simulink model "TSMCDTC"  (R2016b)
settings: Solver=VariableStepAuto  StartTime=0.0  StopTime=1  RelTol=1e-3  EnableMultiTasking=on
model workspace (MAT data in the model file):
  Cf = 1e-05
  J = 0.02
  Lf = 0.005
  Lm = 0.27325
  Lr = 0.289368
  Ls = 0.289368
  P = 4
  Rf = 5
  Rr = 3.3278
  Rs = 4.6
  theta0 = 0
undefined symbols (not defined in the file or in its folder): magnitude
libraries: powerlib x35, simulink x3
settings Model: PauseTimes=0.0143  Creator=yoush  LastModifiedBy=itsys
settings DataIOCC: LimitDataPoints=on  SaveFormat=Array
settings OptimizationCC: LifeSpan=inf
settings DebuggingCC: UnderspecifiedInitializationDetection=Classic  MergeDetectMultiDrivingBlocksExec=none  SolverPrmCheckMsg=warning  AllowSymbolicDim=off  SFUnexpectedBacktrackingDiag=warning  SFNoUnconditionalDefaultTransitionDiag=warning  SFExecutionAtInitializationDiag=none
settings HardwareCC: ProdBitPerPointer=32  ProdBitPerSizeT=32  ProdBitPerPtrDiffT=32  ProdLargestAtomicFloat=None  ProdIntDivRoundTo=Undefined  ProdEndianess=Unspecified  ProdWordSize=32  ProdHWDeviceType=32-bit Generic
settings ModelReferenceCC: PropagateSignalLabelsOutOfModel=off
settings GRTTargetCC: TargetLangStandard=C89/C90 (ANSI)  GeneratePreprocessorConditionals=Disable all
settings ConfigComp: CovMetricSettings=dw  CovHtmlReporting=on  CovSaveCumulativeToWorkspaceVar=on  CovSaveSingleToWorkspaceVar=on  CovExternalEMLEnable=off

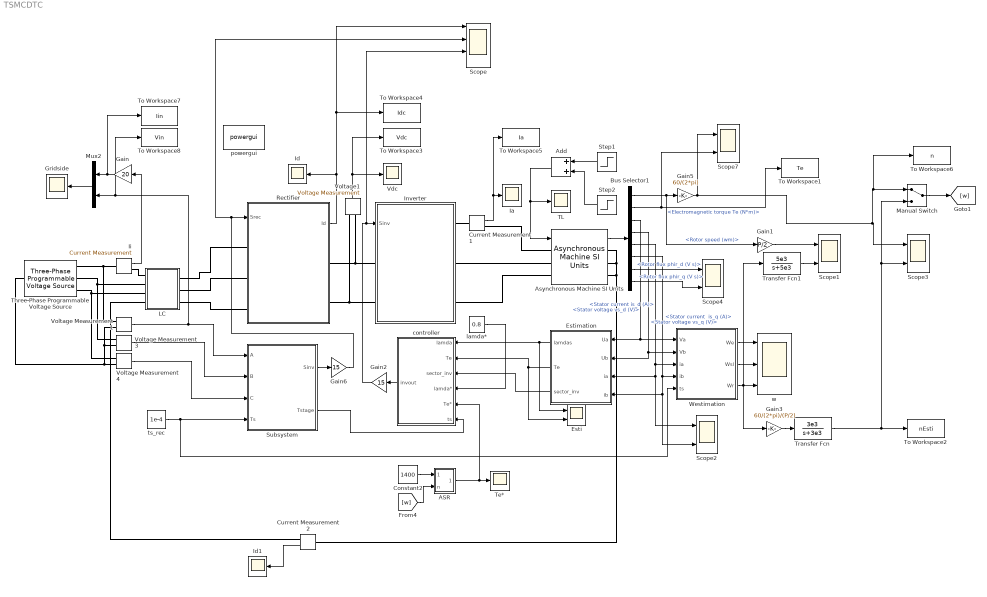
== system TSMCDTC ==
  ASR : Subsystem
  Add : Sum
  Asynchronous Machine SI Units : powerlib/Machines/Asynchronous Machine SI Units  RotorType=Wound  PresetModel=No  MechanicalLoad=Torque Tm  ShowDetailedParameters=on  ReferenceFrame=Stationary  Units=SI  MeasurementBus=off  NominalParameters=[22000 380 50]  Stator=[4.6 0.016118]  Rotor=[3.3278 0.016118]  Cage1=[0.4155 0.002066]  Cage2=[0.4168 0.0003495]  Lm=0.27325  Mechanical=[0.02 0 2]  PolePairs=2  InitialConditions=[ 1 0 0 0 0 0 0 0]  SimulateSaturation=off  Saturation=[14.03593122, 27.81365428, 53.79336849, 72.68890987, 97.98006896, 148.6815601, 215.7428561, 302.9841135, 428.7778367 ; 230, 322, 414, 460, 506, 552, 598, 644, 690]  LoadFlowParameters=1492000  TsPowergui=0  TsBlock=-1  IterativeModel=Trapezoidal non iterative  IterativeDiscreteModel=Trapezoidal non iterative  Pmec=1.492e+006
  Bus Selector1 : BusSelector  OutputSignals="Mechanical.Rotor speed (wm),Mechanical.Electromagnetic torque Te (N*m),Stator measurements.Stator voltage vs_d (V),Stator measurements.Stator voltage vs_q (V),Stator measurements.Stator current is_d (A),Stator measurements.Stator current  is_q (A),Rotor measurements.Rotor flux phir_d (V s),Rotor measurements.Rotor flux phir_q (V s)"
  Constant2 : Constant  Value=1400
  Current Measurement1 : powerlib/Measurements/Current Measurement  PhasorSimulation=off  OutputType=Complex  PSBequivalent=0
  Current Measurement2 : powerlib/Measurements/Current Measurement  PhasorSimulation=off  OutputType=Complex  PSBequivalent=0
  Esti : Scope  NumInputPorts=2
  Estimation : Subsystem
  Gain : Gain  Gain=20
  Gain1 : Gain  Gain=P/2
  Gain2 : Gain  Gain=15
  Gain3 : Gain  Gain=60/(2*pi)/(P/2)
  Gain5 : Gain  Gain=60/(2*pi)
  Gain6 : Gain  Gain=15
  Gridside : Scope
  Ia : Scope
  Id : Scope
  Id1 : Scope
  Ii : powerlib/Measurements/Current Measurement  PhasorSimulation=off  OutputType=Complex  PSBequivalent=0
  Inverter : Subsystem
  LC : Subsystem
  Manual Switch : ManualSwitch
  Mux2 : Mux  Inputs=2
  Rectifier : Subsystem
  Scope : Scope  NumInputPorts=4
  Scope{1..4,7} (5 alike) : Scope  NumInputPorts=2
  Step1 : Step  Time=0.4  After=5  SampleTime=0
  Step2 : Step  Time=0.7  After=5  SampleTime=0
  Subsystem : Subsystem
  TL : Scope
  Te* : Scope
  Three-Phase Programmable Voltage Source : powerlib/Electrical Sources/Three-Phase Programmable Voltage Source  PositiveSequence="[380  0 50]"  VariationEntity=None  VariationType=Table of time-amplitude pairs  VariationTypeAlt=Step  VariationStep=0.5  VariationRate=10  VariationMagnitude=0.3  VariationFrequency=2  VariationTiming=[1 2]  VariationPhaseA=off  Amplitudes=[1 0.8 1.2 1.0]  TimeValues=[0 0.1 0.15 0.2]  HarmonicGeneration=off  HarmonicA=[3 0.2 -25 0]  HarmonicB=[2 0.15 35 2]  Timing="[0.05  3]"  BusType=swing  Pref=0  Qref=0  Qmin=-inf  Qmax=inf
  To Workspace1 : ToWorkspace  VariableName=Te  SaveFormat=Timeseries  SampleTime=-1
  To Workspace2 : ToWorkspace  VariableName=nEsti  SaveFormat=Timeseries  SampleTime=-1
  To Workspace3 : ToWorkspace  VariableName=Vdc  SaveFormat=Timeseries  SampleTime=-1
  To Workspace4 : ToWorkspace  VariableName=Idc  SaveFormat=Timeseries  SampleTime=-1
  To Workspace5 : ToWorkspace  VariableName=Ia  SaveFormat=Timeseries  SampleTime=-1
  To Workspace6 : ToWorkspace  VariableName=n  SaveFormat=Timeseries  SampleTime=-1
  To Workspace7 : ToWorkspace  VariableName=Iin  SaveFormat=Timeseries  SampleTime=-1
  To Workspace8 : ToWorkspace  VariableName=Vin  SaveFormat=Timeseries  SampleTime=-1
  Transfer Fcn : TransferFcn  Numerator=[3e3]  Denominator=[1 3e3]
  Transfer Fcn1 : TransferFcn  Numerator=[5e3]  Denominator=[1 5e3]
  Vdc : Scope
  Voltage Measurement1 : powerlib/Measurements/Voltage Measurement  PhasorSimulation=off  OutputType=Complex  PSBequivalent=0
  Voltage Measurement3 : powerlib/Measurements/Voltage Measurement  PhasorSimulation=off  OutputType=Complex  PSBequivalent=0
  Voltage Measurement4 : powerlib/Measurements/Voltage Measurement  PhasorSimulation=off  OutputType=Complex  PSBequivalent=0
  Voltage1 : powerlib/Measurements/Voltage Measurement  PhasorSimulation=off  OutputType=Complex  PSBequivalent=0
  Westimation : Subsystem
  controller : Subsystem
  lamda* : Constant  Value=0.8
  powergui : powerlib/powergui  Priority=1  SimulationMode=Continuous  SolverType=Tustin  SampleTime=5e-7  frequency=60  SPID=off  DisableSnubberDevices=off  DisableRonSwitches=off  DisableVfSwitches=off  SwTol=0  DisplayEquations=off  Interpol=off  ExternalGateDelay=off  methode=off  Ts=0  FunctionMessages=off  echomessages=off  HookPort=off  EnableUseOfTLC=off  x0status=blocks  frequencyindice=50  Pbase=100e6  ErrMax=1e-4  Iterations=50  UnitsV=kV  UnitsW=MW  buscounter=0  RestoreLinks=warning  ResistiveCurrentMeasurement=off  Frange=[0:2:500]  Ylog=off  Xlog=on  ShowGrid=off  save=off  variable=ZData  structure=input  ZoomFFT=off  StartTime=0.5  cycles=5  DisplayStyle=1  fundamental=50  FreqAxis=off  MaxFrequency=10000  frequencyindicesteady=1  RmsSteady=1  display=off
  ts_rec : Constant  Value=1e-4
  w : Scope  NumInputPorts=3
  wires:
  Current Measurement1/1 -> To Workspace5/1, Ia/1
  Asynchronous Machine SI Units/1 -> Bus Selector1/1
  Bus Selector1/2 -> Scope7/2, To Workspace1/1  "<Electromagnetic torque Te (N*m)>"
  Bus Selector1/1 -> Gain1/1, Gain5/1  "<Rotor speed (wm)>"
  Bus Selector1/3 -> Estimation/1(Ua), Westimation/1(Va)  "<Stator voltage vs_d (V)>"
  Step1/1 -> Add/1
  Step2/1 -> Add/2
  Add/1 -> Asynchronous Machine SI Units/1, TL/1
  lamda*/1 -> controller/4(lamda*)
  controller/1(invout) -> Gain2/1
  Gain5/1 -> To Workspace6/1, Manual Switch/1, Scope3/1, Scope7/1
  Gain6/1 -> Scope/2, Rectifier/1(Srec)
  Rectifier/1(Id) -> Scope/1, To Workspace4/1, Id/1
  Gain2/1 -> Scope/3, Inverter/1(Sinv)
  Westimation/1(We) -> w/1
  Westimation/2(Wsl) -> w/2
  Bus Selector1/4 -> Westimation/2(Vb), Estimation/2(Ub)  "<Stator voltage vs_q (V)>"
  Bus Selector1/5 -> Westimation/3(ia), Scope2/1, Estimation/3(ia)  "<Stator current is_d (A)>"
  Bus Selector1/6 -> Westimation/4(ib), Scope2/2, Estimation/4(ib)  "<Stator current  is_q (A)>"
  Estimation/1(lamdas) -> Esti/1, controller/1(lamda)
  Estimation/2(Te) -> Esti/2, controller/2(Te)
  Estimation/3(sector_inv) -> controller/3(sector_inv)
  Voltage Measurement1/1 -> To Workspace8/1, Mux2/2, Subsystem/1(A)
  Voltage Measurement3/1 -> Subsystem/2(B)
  Voltage Measurement4/1 -> Subsystem/3(C)
  Subsystem/1(Sinv) -> Gain6/1
  Voltage1/1 -> Vdc/1, To Workspace3/1
  Mux2/1 -> Gridside/1
  Ii/1 -> Gain/1
  Gain1/1 -> Scope1/1
  Gain3/1 -> Transfer Fcn/1
  Westimation/3(Wr) -> Transfer Fcn1/1, Gain3/1, w/3
  Transfer Fcn1/1 -> Scope1/2
  Transfer Fcn/1 -> To Workspace2/1, Manual Switch/2, Scope3/2
  Manual Switch/1 -> [w]
  Bus Selector1/7 -> Scope4/1  "<Rotor flux phir_d (V s)>"
  Bus Selector1/8 -> Scope4/2  "<Rotor flux phir_q (V s)>"
  ASR/1(Te*) -> Te*/1, controller/5(Te*)
  Constant2/1 -> ASR/1(n*)
  [w] -> ASR/2(n)
  ts_rec/1 -> Westimation/5(ts), Subsystem/4(Ts)
  Subsystem/2(Tstage) -> controller/6(ts)
  Gain/1 -> To Workspace7/1, Mux2/1
  Current Measurement2/1 -> Id1/1
  connections:
  Voltage Measurement1/LConn1 -- Three-Phase Programmable Voltage Source/RConn1 -- Ii/LConn1
  Three-Phase Programmable Voltage Source/LConn1 -- Voltage Measurement1/LConn2 -- Voltage Measurement3/LConn2 -- Voltage Measurement4/LConn2
  Current Measurement1/RConn1 -- Asynchronous Machine SI Units/LConn1
  Current Measurement1/LConn1 -- Inverter/RConn1
  Asynchronous Machine SI Units/LConn2 -- Inverter/RConn2
  Asynchronous Machine SI Units/LConn3 -- Inverter/RConn3
  Rectifier/RConn1 -- Inverter/LConn1 -- Voltage1/LConn1
  Rectifier/RConn2 -- Inverter/LConn2 -- Voltage1/LConn2
  Voltage Measurement3/LConn1 -- Three-Phase Programmable Voltage Source/RConn2 -- LC/LConn2
  Three-Phase Programmable Voltage Source/RConn3 -- LC/LConn3 -- Voltage Measurement4/LConn1
  LC/LConn1 -- Ii/RConn1
  LC/RConn1 -- Rectifier/LConn1
  LC/RConn2 -- Rectifier/LConn2
  LC/RConn3 -- Rectifier/LConn3
  Asynchronous Machine SI Units/RConn2 -- Current Measurement2/LConn1 -- Asynchronous Machine SI Units/RConn3 -- Asynchronous Machine SI Units/RConn1
  Current Measurement2/RConn1 -- LC/LConn4

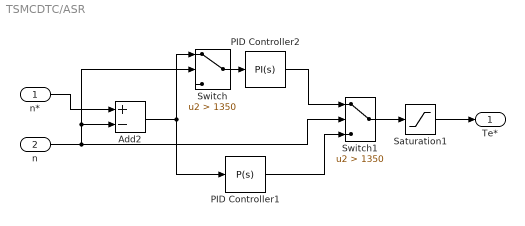
== system TSMCDTC/ASR ==
  n* : Inport
  n : Inport  Port=2
  Add2 : Sum  Inputs=+-
  PID Controller1 : simulink/Continuous/PID Controller  Controller=P  TimeDomain=Continuous-time  SampleTime=-1  IntegratorMethod=Forward Euler  FilterMethod=Forward Euler  Form=Parallel  UseFilter=on  ControllerParametersSource=internal  P=1  I=0  D=0  N=100  InitialConditionSource=internal  InitialConditionForIntegrator=0  InitialConditionForFilter=0  ExternalReset=none  LimitOutput=off  UpperSaturationLimit=inf  LowerSaturationLimit=-inf  LinearizeAsGain=on  AntiWindupMode=none  Kb=1  TrackingMode=off  Kt=1  PParamMin=[]  PParamMax=[]  IParamMin=[]  IParamMax=[]  DParamMin=[]  DParamMax=[]  NParamMin=[]  NParamMax=[]  KbParamMin=[]  KbParamMax=[]  KtParamMin=[]  KtParamMax=[]  POutMin=[]  POutMax=[]  IOutMin=[]  IOutMax=[]  DOutMin=[]  DOutMax=[]  NOutMin=[]  NOutMax=[]  KbOutMin=[]  KbOutMax=[]  KtOutMin=[]  KtOutMax=[]  IntegratorOutMin=[]  IntegratorOutMax=[]  FilterOutMin=[]  FilterOutMax=[]  SumOutMin=[]  SumOutMax=[]  SumI1OutMin=[]  SumI1OutMax=[]  SumI2OutMin=[]  SumI2OutMax=[]  SumI3OutMin=[]  SumI3OutMax=[]  SumDOutMin=[]  SumDOutMax=[]  SaturationOutMin=[]  SaturationOutMax=[]  IntegratorContinuousStateAttributes=''  IntegratorStateMustResolveToSignalObject=off  IntegratorRTWStateStorageClass=Auto  FilterContinuousStateAttributes=''  FilterStateMustResolveToSignalObject=off  FilterRTWStateStorageClass=Auto  DifferentiatorICPrevScaledInput=0  DifferentiatorOutMin=[]  DifferentiatorOutMax=[]
  PID Controller2 : simulink/Continuous/PID Controller  Controller=PI  TimeDomain=Continuous-time  SampleTime=-1  IntegratorMethod=Forward Euler  FilterMethod=Forward Euler  Form=Parallel  UseFilter=on  ControllerParametersSource=internal  P=0.3  I=30  D=0  N=100  InitialConditionSource=internal  InitialConditionForIntegrator=0  InitialConditionForFilter=0  ExternalReset=none  LimitOutput=off  UpperSaturationLimit=inf  LowerSaturationLimit=-inf  LinearizeAsGain=on  AntiWindupMode=none  Kb=1  TrackingMode=off  Kt=1  PParamMin=[]  PParamMax=[]  IParamMin=[]  IParamMax=[]  DParamMin=[]  DParamMax=[]  NParamMin=[]  NParamMax=[]  KbParamMin=[]  KbParamMax=[]  KtParamMin=[]  KtParamMax=[]  POutMin=[]  POutMax=[]  IOutMin=[]  IOutMax=[]  DOutMin=[]  DOutMax=[]  NOutMin=[]  NOutMax=[]  KbOutMin=[]  KbOutMax=[]  KtOutMin=[]  KtOutMax=[]  IntegratorOutMin=[]  IntegratorOutMax=[]  FilterOutMin=[]  FilterOutMax=[]  SumOutMin=[]  SumOutMax=[]  SumI1OutMin=[]  SumI1OutMax=[]  SumI2OutMin=[]  SumI2OutMax=[]  SumI3OutMin=[]  SumI3OutMax=[]  SumDOutMin=[]  SumDOutMax=[]  SaturationOutMin=[]  SaturationOutMax=[]  IntegratorContinuousStateAttributes=''  IntegratorStateMustResolveToSignalObject=off  IntegratorRTWStateStorageClass=Auto  FilterContinuousStateAttributes=''  FilterStateMustResolveToSignalObject=off  FilterRTWStateStorageClass=Auto  DifferentiatorICPrevScaledInput=0  DifferentiatorOutMin=[]  DifferentiatorOutMax=[]
  Saturation1 : Saturate  UpperLimit=15  LowerLimit=-15
  Switch : Switch  Criteria=u2 > Threshold  Threshold=1350
  Switch1 : Switch  Criteria=u2 > Threshold  Threshold=1350
  Te* : Outport
  wires:
  Saturation1/1 -> Te*/1
  PID Controller1/1 -> Switch1/3
  Switch1/1 -> Saturation1/1
  PID Controller2/1 -> Switch1/1
  Switch/1 -> PID Controller2/1
  Add2/1 -> PID Controller1/1, Switch/1
  n*/1 -> Add2/1
  n/1 -> Switch1/2, Switch/2, Add2/2

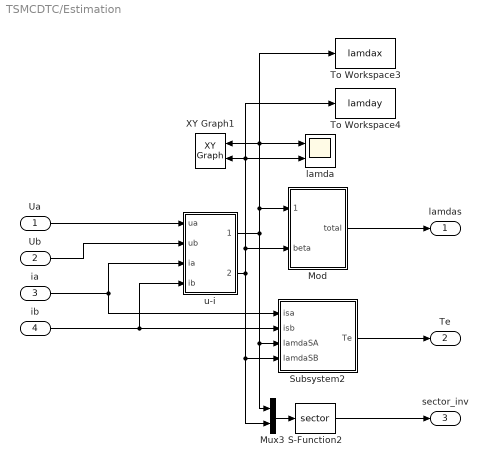
== system TSMCDTC/Estimation ==
  Ua : Inport
  Ub : Inport  Port=2
  ia : Inport  Port=3
  ib : Inport  Port=4
  Mod : Subsystem
  Mux3 : Mux  Inputs=2
  S-Function2 : S-Function  FunctionName=sector  SFunctionDeploymentMode=off  EnableBusSupport=off
  Subsystem2 : Subsystem
  To Workspace3 : ToWorkspace  VariableName=lamdax  SaveFormat=Timeseries  SampleTime=-1
  To Workspace4 : ToWorkspace  VariableName=lamday  SaveFormat=Timeseries  SampleTime=-1
  XY Graph1 : simulink/Sinks/XY Graph  xmin=-1.5  xmax=1.5  ymin=-1.5  ymax=1.5  st=-1
  lamda : Scope  NumInputPorts=2
  u-i : Subsystem
  lamdas : Outport
  Te : Outport  Port=2
  sector_inv : Outport  Port=3
  wires:
  u-i/1(lamdaSA) -> Mux3/1, Subsystem2/3(lamdaSA), To Workspace3/1, lamda/1, XY Graph1/1, Mod/1(alpha)
  u-i/2(lamdaSB) -> Mux3/2, Subsystem2/4(lamdaSB), To Workspace4/1, lamda/2, XY Graph1/2, Mod/2(beta)
  Mux3/1 -> S-Function2/1
  Ua/1 -> u-i/1(ua)
  Ub/1 -> u-i/2(ub)
  ia/1 -> u-i/3(ia), Subsystem2/1(isa)
  ib/1 -> u-i/4(ib), Subsystem2/2(isb)
  S-Function2/1 -> sector_inv/1
  Subsystem2/1(Te) -> Te/1
  Mod/1(total) -> lamdas/1

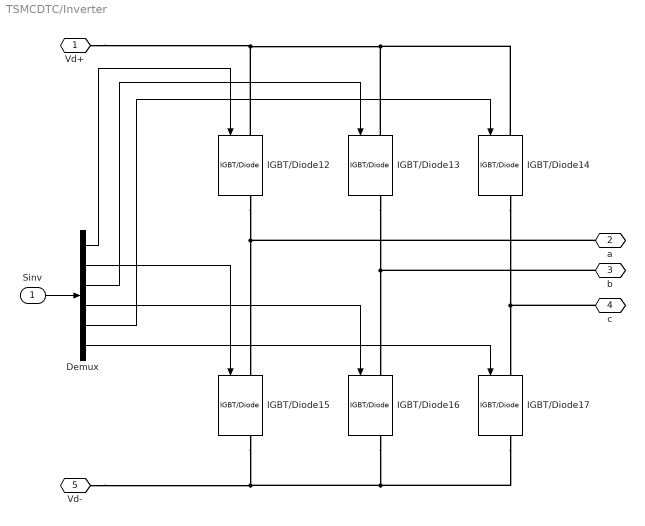
== system TSMCDTC/Inverter ==
  Sinv : Inport
  Demux : Demux  Outputs=6
  IGBT/Diode{12..17} (6 alike) : powerlib/Power Electronics/IGBT//Diode  Ron=1e-3  Rs=1e5  Cs=inf  Measurements=on
  Vd+ : PMIOPort  Port=1  Side=Left
  a : PMIOPort  Port=2  Side=Right
  b : PMIOPort  Port=3  Side=Right
  c : PMIOPort  Port=4  Side=Right
  Vd- : PMIOPort  Port=5  Side=Left
  wires:
  Demux/5 -> IGBT/Diode14/1
  Demux/4 -> IGBT/Diode16/1
  Demux/3 -> IGBT/Diode13/1
  Demux/6 -> IGBT/Diode17/1
  Demux/1 -> IGBT/Diode12/1
  Sinv/1 -> Demux/1
  Demux/2 -> IGBT/Diode15/1
  connections:
  IGBT/Diode12/RConn1 -- IGBT/Diode15/LConn1 -- a/RConn1
  IGBT/Diode13/RConn1 -- IGBT/Diode16/LConn1 -- b/RConn1
  IGBT/Diode14/RConn1 -- IGBT/Diode17/LConn1 -- c/RConn1
  IGBT/Diode17/RConn1 -- IGBT/Diode16/RConn1 -- Vd-/RConn1 -- IGBT/Diode15/RConn1
  IGBT/Diode12/LConn1 -- Vd+/RConn1 -- IGBT/Diode13/LConn1 -- IGBT/Diode14/LConn1

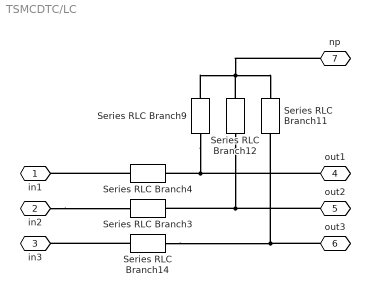
== system TSMCDTC/LC ==
  Series RLC Branch11 : powerlib/Elements/Series RLC Branch  LConnTagsString=__new0  RConnTagsString=__new0  BranchType=C  Resistance=1  Inductance=0.5e-3  SetiL0=off  InitialCurrent=0  Capacitance=Cf  Setx0=off  InitialVoltage=0  Measurements=None
  Series RLC Branch12 : powerlib/Elements/Series RLC Branch  LConnTagsString=__new0  RConnTagsString=__new0  BranchType=C  Resistance=1  Inductance=0.5e-3  SetiL0=off  InitialCurrent=0  Capacitance=Cf  Setx0=off  InitialVoltage=0  Measurements=None
  Series RLC Branch14 : powerlib/Elements/Series RLC Branch  LConnTagsString=__new0  RConnTagsString=__new0  BranchType=RL  Resistance=Rf  Inductance=Lf  SetiL0=off  InitialCurrent=0  Capacitance=1e-6  Setx0=off  InitialVoltage=0  Measurements=None
  Series RLC Branch3 : powerlib/Elements/Series RLC Branch  LConnTagsString=__new0  RConnTagsString=__new0  BranchType=RL  Resistance=Rf  Inductance=Lf  SetiL0=off  InitialCurrent=0  Capacitance=1e-6  Setx0=off  InitialVoltage=0  Measurements=None
  Series RLC Branch4 : powerlib/Elements/Series RLC Branch  LConnTagsString=__new0  RConnTagsString=__new0  BranchType=RL  Resistance=Rf  Inductance=Lf  SetiL0=off  InitialCurrent=0  Capacitance=1e-6  Setx0=off  InitialVoltage=0  Measurements=None
  Series RLC Branch9 : powerlib/Elements/Series RLC Branch  LConnTagsString=__new0  RConnTagsString=__new0  BranchType=C  Resistance=1  Inductance=0.5e-3  SetiL0=off  InitialCurrent=0  Capacitance=Cf  Setx0=off  InitialVoltage=0  Measurements=None
  in1 : PMIOPort  Port=1  Side=Left
  in2 : PMIOPort  Port=2  Side=Left
  in3 : PMIOPort  Port=3  Side=Left
  out1 : PMIOPort  Port=4  Side=Right
  out2 : PMIOPort  Port=5  Side=Right
  out3 : PMIOPort  Port=6  Side=Right
  np : PMIOPort  Port=7  Side=Left
  connections:
  Series RLC Branch4/LConn1 -- in1/RConn1
  Series RLC Branch14/LConn1 -- in3/RConn1
  in2/RConn1 -- Series RLC Branch3/LConn1
  Series RLC Branch9/RConn1 -- np/RConn1 -- Series RLC Branch12/RConn1 -- Series RLC Branch11/RConn1
  out1/RConn1 -- Series RLC Branch9/LConn1 -- Series RLC Branch4/RConn1
  out2/RConn1 -- Series RLC Branch12/LConn1 -- Series RLC Branch3/RConn1
  Series RLC Branch14/RConn1 -- out3/RConn1 -- Series RLC Branch11/LConn1

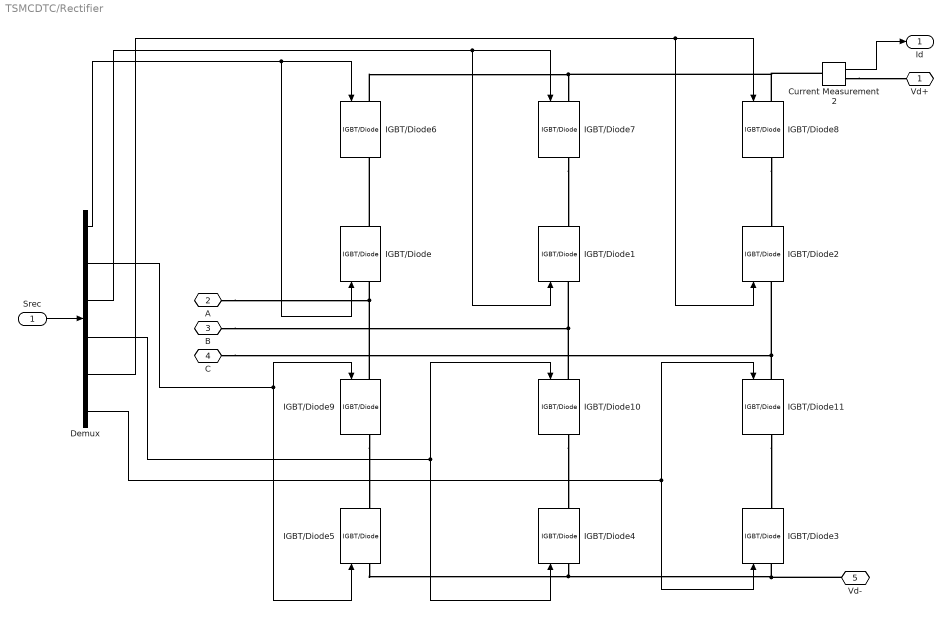
== system TSMCDTC/Rectifier ==
  Srec : Inport
  Current Measurement2 : powerlib/Measurements/Current Measurement  PhasorSimulation=off  OutputType=Complex  PSBequivalent=0
  Demux : Demux  Outputs=6
  IGBT/Diode{,1..11} (12 alike) : powerlib/Power Electronics/IGBT//Diode  Ron=1e-3  Rs=1e5  Cs=inf  Measurements=on
  Vd+ : PMIOPort  Port=1  Side=Right
  A : PMIOPort  Port=2  Side=Left
  B : PMIOPort  Port=3  Side=Left
  "C " : PMIOPort  Port=4  Side=Left
  Vd- : PMIOPort  Port=5  Side=Right
  Id : Outport
  wires:
  Srec/1 -> Demux/1
  Demux/1 -> IGBT/Diode/1, IGBT/Diode6/1
  Demux/2 -> IGBT/Diode5/1, IGBT/Diode9/1
  Demux/3 -> IGBT/Diode1/1, IGBT/Diode7/1
  Demux/5 -> IGBT/Diode8/1, IGBT/Diode2/1
  Demux/4 -> IGBT/Diode10/1, IGBT/Diode4/1
  Demux/6 -> IGBT/Diode3/1, IGBT/Diode11/1
  Current Measurement2/1 -> Id/1
  connections:
  IGBT/Diode11/RConn1 -- IGBT/Diode3/RConn1
  IGBT/Diode10/RConn1 -- IGBT/Diode4/RConn1
  IGBT/Diode8/RConn1 -- IGBT/Diode2/RConn1
  IGBT/Diode9/RConn1 -- IGBT/Diode5/RConn1
  IGBT/Diode9/LConn1 -- A/RConn1 -- IGBT/Diode/LConn1
  IGBT/Diode6/LConn1 -- IGBT/Diode8/LConn1 -- Current Measurement2/LConn1 -- IGBT/Diode7/LConn1
  IGBT/Diode7/RConn1 -- IGBT/Diode1/RConn1
  IGBT/Diode/RConn1 -- IGBT/Diode6/RConn1
  IGBT/Diode10/LConn1 -- B/RConn1 -- IGBT/Diode1/LConn1
  IGBT/Diode11/LConn1 -- "C "/RConn1 -- IGBT/Diode2/LConn1
  IGBT/Diode5/LConn1 -- IGBT/Diode4/LConn1 -- Vd-/RConn1 -- IGBT/Diode3/LConn1
  Current Measurement2/RConn1 -- Vd+/RConn1

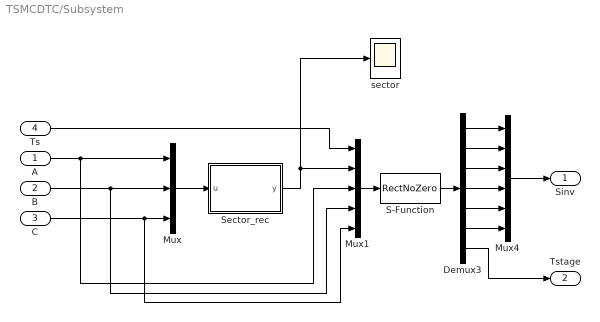
== system TSMCDTC/Subsystem ==
  A : Inport
  B : Inport  Port=2
  C : Inport  Port=3
  Ts : Inport  Port=4
  Demux3 : Demux  Outputs=7
  Mux : Mux  Inputs=3
  Mux1 : Mux  Inputs=5
  Mux4 : Mux  Inputs=6
  S-Function : S-Function  FunctionName=RectNoZero  SFunctionDeploymentMode=off  EnableBusSupport=off
  Sector_rec : MATLAB Function  TreatAsAtomicUnit=on
  sector : Scope
  Sinv : Outport
  Tstage : Outport  Port=2
  wires:
  B/1 -> Mux/2, Mux1/4
  Mux/1 -> Sector_rec/1(u)
  A/1 -> Mux/1, Mux1/3
  Sector_rec/1(y) -> Mux1/2, sector/1
  C/1 -> Mux1/5, Mux/3
  Demux3/5 -> Mux4/5
  Demux3/6 -> Mux4/6
  Demux3/2 -> Mux4/2
  Demux3/1 -> Mux4/1
  Mux4/1 -> Sinv/1
  S-Function/1 -> Demux3/1
  Demux3/4 -> Mux4/4
  Demux3/3 -> Mux4/3
  Mux1/1 -> S-Function/1
  Ts/1 -> Mux1/1
  Demux3/7 -> Tstage/1

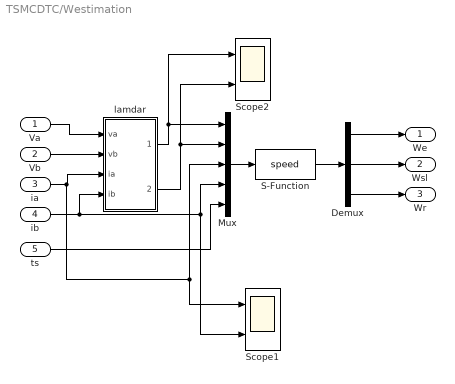
== system TSMCDTC/Westimation ==
  Va : Inport
  Vb : Inport  Port=2
  ia : Inport  Port=3
  ib : Inport  Port=4
  ts : Inport  Port=5
  Demux : Demux  Outputs=3
  Mux : Mux  Inputs=5
  S-Function : S-Function  FunctionName=speed  SFunctionDeploymentMode=off  EnableBusSupport=off
  Scope1 : Scope  NumInputPorts=2
  Scope2 : Scope  NumInputPorts=2
  lamdar : Subsystem
  We : Outport
  Wsl : Outport  Port=2
  Wr : Outport  Port=3
  wires:
  ts/1 -> Mux/5
  lamdar/2(lamdarb) -> Scope2/2, Mux/2
  lamdar/1(lamdara) -> Scope2/1, Mux/1
  Demux/3 -> Wr/1
  Demux/2 -> Wsl/1
  Demux/1 -> We/1
  S-Function/1 -> Demux/1
  Mux/1 -> S-Function/1
  Va/1 -> lamdar/1(va)
  Vb/1 -> lamdar/2(vb)
  ia/1 -> Scope1/1, Mux/3, lamdar/3(ia)
  ib/1 -> Scope1/2, Mux/4, lamdar/4(ib)

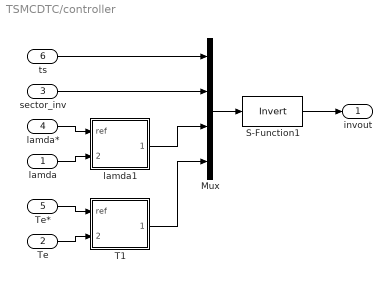
== system TSMCDTC/controller ==
  lamda : Inport
  Te : Inport  Port=2
  sector_inv : Inport  Port=3
  lamda* : Inport  Port=4
  Te* : Inport  Port=5
  ts : Inport  Port=6
  Mux : Mux
  S-Function1 : S-Function  FunctionName=Invert  SFunctionDeploymentMode=off  EnableBusSupport=off
  T1 : Subsystem
  lamda1 : Subsystem
  invout : Outport
  wires:
  Te*/1 -> T1/1(ref)
  Te/1 -> T1/2(measure)
  lamda*/1 -> lamda1/1(ref)
  lamda/1 -> lamda1/2(measure)
  S-Function1/1 -> invout/1
  Mux/1 -> S-Function1/1
  ts/1 -> Mux/1
  sector_inv/1 -> Mux/2
  lamda1/1(Out1) -> Mux/3
  T1/1(Out1) -> Mux/4

== system TSMCDTC/Estimation/Mod ==
  alpha : Inport
  beta : Inport  Port=2
  Add : Sum
  Math Function : Math  Operator=magnitude^2  SaturateOnIntegerOverflow=on
  Math Function1 : Math  Operator=magnitude^2  SaturateOnIntegerOverflow=on
  Sqrt : Sqrt  SaturateOnIntegerOverflow=on
  total : Outport
  wires:
  alpha/1 -> Math Function/1
  beta/1 -> Math Function1/1
  Math Function/1 -> Add/1
  Math Function1/1 -> Add/2
  Add/1 -> Sqrt/1
  Sqrt/1 -> total/1

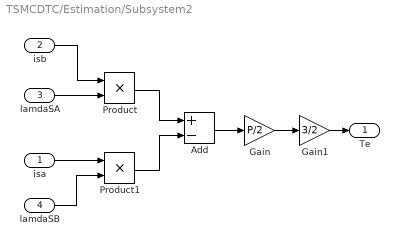
== system TSMCDTC/Estimation/Subsystem2 ==
  isa : Inport
  isb : Inport  Port=2
  lamdaSA : Inport  Port=3
  lamdaSB : Inport  Port=4
  Add : Sum  Inputs=+-
  Gain : Gain  Gain=P/2
  Gain1 : Gain  Gain=3/2
  Product : Product
  Product1 : Product
  Te : Outport
  wires:
  Add/1 -> Gain/1
  Product/1 -> Add/1
  Product1/1 -> Add/2
  lamdaSA/1 -> Product/2
  isb/1 -> Product/1
  isa/1 -> Product1/1
  lamdaSB/1 -> Product1/2
  Gain/1 -> Gain1/1
  Gain1/1 -> Te/1

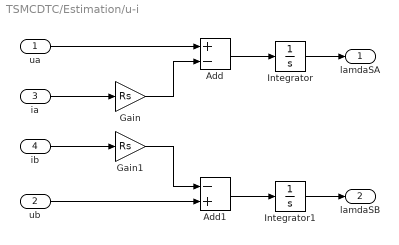
== system TSMCDTC/Estimation/u-i ==
  ua : Inport
  ub : Inport  Port=2
  ia : Inport  Port=3
  ib : Inport  Port=4
  Add : Sum  Inputs=+-
  Add1 : Sum  Inputs=-+
  Gain : Gain  Gain=Rs
  Gain1 : Gain  Gain=Rs
  Integrator : Integrator
  Integrator1 : Integrator
  lamdaSA : Outport
  lamdaSB : Outport  Port=2
  wires:
  ib/1 -> Gain1/1
  ia/1 -> Gain/1
  Gain/1 -> Add/2
  ua/1 -> Add/1
  ub/1 -> Add1/2
  Gain1/1 -> Add1/1
  Add/1 -> Integrator/1
  Add1/1 -> Integrator1/1
  Integrator1/1 -> lamdaSB/1
  Integrator/1 -> lamdaSA/1

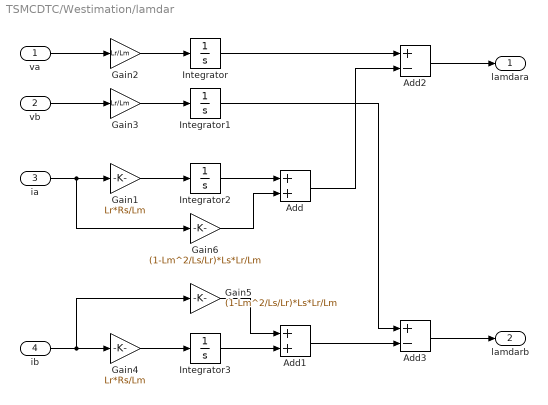
== system TSMCDTC/Westimation/lamdar ==
  va : Inport
  vb : Inport  Port=2
  ia : Inport  Port=3
  ib : Inport  Port=4
  Add : Sum
  Add1 : Sum
  Add2 : Sum  Inputs=+-
  Add3 : Sum  Inputs=+-
  Gain1 : Gain  Gain=Lr*Rs/Lm
  Gain2 : Gain  Gain=Lr/Lm
  Gain3 : Gain  Gain=Lr/Lm
  Gain4 : Gain  Gain=Lr*Rs/Lm
  Gain5 : Gain  Gain=(1-Lm^2/Ls/Lr)*Ls*Lr/Lm
  Gain6 : Gain  Gain=(1-Lm^2/Ls/Lr)*Ls*Lr/Lm
  Integrator{,1..3} (4 alike) : Integrator
  lamdara : Outport
  lamdarb : Outport  Port=2
  wires:
  Add3/1 -> lamdarb/1
  Integrator1/1 -> Add3/1
  Add1/1 -> Add3/2
  Add2/1 -> lamdara/1
  Add/1 -> Add2/2
  Integrator/1 -> Add2/1
  Gain5/1 -> Add1/1
  Integrator3/1 -> Add1/2
  Gain6/1 -> Add/2
  Integrator2/1 -> Add/1
  Gain4/1 -> Integrator3/1
  ib/1 -> Gain4/1, Gain5/1
  Gain1/1 -> Integrator2/1
  ia/1 -> Gain1/1, Gain6/1
  Gain3/1 -> Integrator1/1
  vb/1 -> Gain3/1
  Gain2/1 -> Integrator/1
  va/1 -> Gain2/1

== system TSMCDTC/controller/T1 ==
  ref : Inport
  measure : Inport  Port=2
  Add : Sum  Inputs=+-
  Add1 : Sum
  Relay : Relay  OnSwitchValue=0.1  OffSwitchValue=-0.1
  Relay1 : Relay  OnSwitchValue=0  OffSwitchValue=0  OnOutputValue=0.5  OffOutputValue=-0.5
  Scope : Scope
  Out1 : Outport
  wires:
  Add/1 -> Relay/1
  ref/1 -> Add/1
  measure/1 -> Add/2
  Relay/1 -> Scope/1, Out1/1

== system TSMCDTC/controller/lamda1 ==
  ref : Inport
  measure : Inport  Port=2
  Add : Sum  Inputs=+-
  Relay : Relay  OnSwitchValue=0.01  OffSwitchValue=-0.01
  Out1 : Outport
  wires:
  Relay/1 -> Out1/1
  Add/1 -> Relay/1
  ref/1 -> Add/1
  measure/1 -> Add/2

== matlab function TSMCDTC/Subsystem/Sector_rec ==
  data: u input; y output
function y = fcn(u)
if (u(1) > 0 && u(2) < 0 && u(3) <= 0)
    y = 1;
elseif (u(1) > 0 && u(2) >= 0 && u(3) < 0)
    y = 2;
elseif (u(1) <= 0 && u(2) > 0 && u(3) < 0)
    y = 3;
elseif (u(1) < 0 && u(2) > 0 && u(3) >= 0)
    y = 4;
elseif (u(1) < 0 && u(2) <= 0 && u(3) > 0)
    y = 5;
else
    y = 6;
end
